simulink model "cl_pi"  (R2012b)
settings: Solver=FixedStepDiscrete  StartTime=0.0  StopTime=20.0  RelTol=1e-3
values from neighbouring files (symbols this model uses):
  A = reshape(A_w(i, :, :), 4, 4)    [tune_pi.m]
  A_e = reshape(A_e_w(i, :, :), 4, 4)    [tune_pi.m]
  B = reshape(B_c_w(i, :, :), 4, 1)    [tune_pi.m]
  B_e = reshape(B_e_w(i, :, :), 4, 3)    [tune_pi.m]
  C_m = reshape(C_m_w(i, :, :), 2, 4)    [tune_pi.m]
  C_z = reshape(C_z_w(i, :, :), 1, 4)    [tune_pi.m]
  dt = 0.005    [tune_pi.m]
  K_c = reshape(K_c_w(i, :, :), 1, 4)    [tune_pi.m]
  pid_ss = ss(C_pi)    [tune_pi.m]
  x0 = zeros(4, 1)    [tune_pi.m]
settings Model: Creator=hazelnusse  LastModifiedBy=hazelnusse
settings DataIOCC: LimitDataPoints=off  SaveOutput=off  TimeSaveName=t

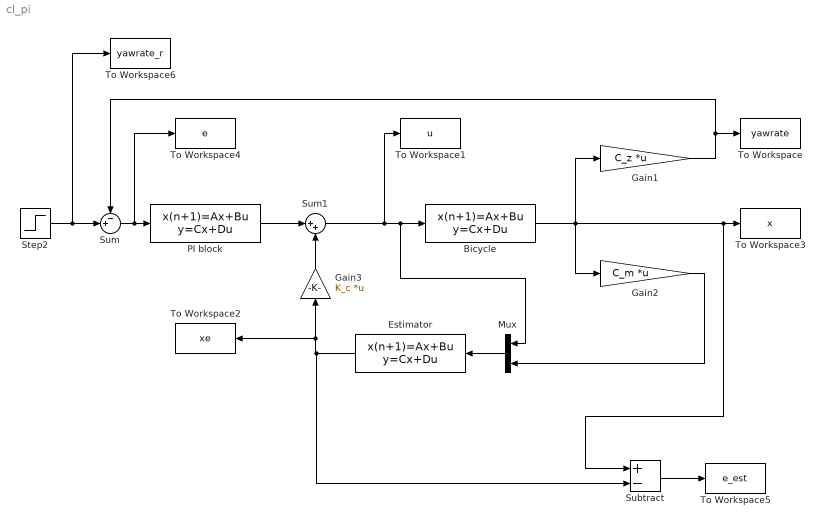
== system cl_pi ==
  Bicycle : DiscreteStateSpace  A=A  B=B  C=eye(4)  D=zeros(4, 1)  X0=x0  SampleTime=dt
  Estimator : DiscreteStateSpace  A=A_e  B=B_e  C=eye(4)  D=zeros(4, 3)  SampleTime=dt
  Gain1 : Gain  Gain=C_z  Multiplication=Matrix(K*u)  SampleTime=dt
  Gain2 : Gain  Gain=C_m  Multiplication=Matrix(K*u)  SampleTime=dt
  Gain3 : Gain  Gain=K_c  Multiplication=Matrix(K*u)
  Mux : Mux  Inputs=2
  PI block : DiscreteStateSpace  A=pid_ss.a  B=pid_ss.b  C=pid_ss.c  D=pid_ss.d  SampleTime=dt
  Step2 : Step  Time=0  After=45*pi/180.  SampleTime=dt
  Subtract : Sum  Inputs=+-
  Sum : Sum  Inputs=-+|
  Sum1 : Sum  Inputs=|++
  To Workspace : ToWorkspace  VariableName=yawrate  SampleTime=-1
  To Workspace1 : ToWorkspace  VariableName=u  SampleTime=dt
  To Workspace2 : ToWorkspace  VariableName=xe  SampleTime=dt
  To Workspace3 : ToWorkspace  VariableName=x  SampleTime=dt
  To Workspace4 : ToWorkspace  VariableName=e  SampleTime=dt
  To Workspace5 : ToWorkspace  VariableName=e_est  SampleTime=dt
  To Workspace6 : ToWorkspace  VariableName=yawrate_r  SampleTime=-1
  wires:
  PI block/1 -> Sum1/1
  Sum/1 -> To Workspace4/1, PI block/1
  Step2/1 -> To Workspace6/1, Sum/2
  Bicycle/1 -> Subtract/1, To Workspace3/1, Gain2/1, Gain1/1
  Gain1/1 -> Sum/1, To Workspace/1
  Sum1/1 -> To Workspace1/1, Bicycle/1, Mux/1
  Gain2/1 -> Mux/2
  Estimator/1 -> Subtract/2, To Workspace2/1, Gain3/1
  Gain3/1 -> Sum1/2
  Mux/1 -> Estimator/1
  Subtract/1 -> To Workspace5/1
